simulink model "horn"  (Simulink 7.8)
settings: Solver=ode45  StartTime=0.0  StopTime=1000  RelTol=1e-3
undefined symbols (not defined in the file): magnitude
libraries: simulink x8
settings Model: Creator=ranasa1  LastModifiedBy=ranasa1

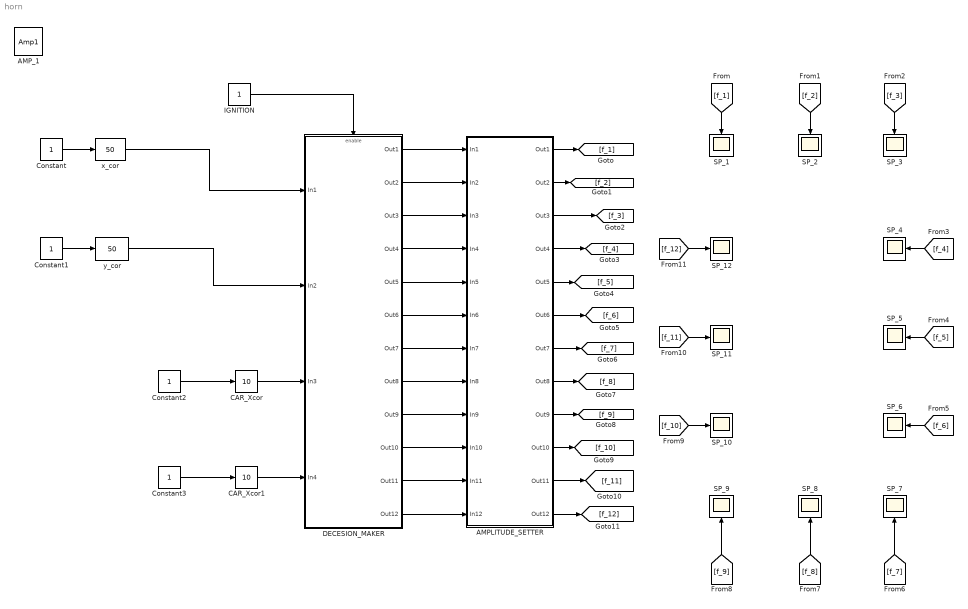
== system horn ==
  AMPLITUDE_SETTER : Subsystem  TreatAsAtomicUnit=on
      settings: RTWFcnNameOpts=Use subsystem name  RTWFileNameOpts=Use function name
  AMP_1 : DataStoreMemory  DataStoreName=Amp1  ReadBeforeWriteMsg=warning  WriteAfterWriteMsg=warning  WriteAfterReadMsg=warning  mask(TL_DataStoreMemory){data={'date',736152.61579912039}}
      settings: CopyFcn=if exist('tl_reset_reviewflag') == 2, tl_reset_reviewflag(gcbh); end  DeleteFcn=if exist('delete_tlblock','file')==2,delete_tlblock(gcbh);end  NameChangeFcn=if exist('rename_tlblock','file')==2,rename_tlblock(gcbh);end  OpenFcn=if exist('tl_open_blockdlg','file')==2,tl_open_blockdlg(gcbh);else,open_system(gcbh,'parameter');end
      mask Help: eval(['if exist(''tl_online_help'',''file'') == 2, tl_online_help(''Topic'',''TL_DataStoreMemory''),else, web([''jar:file:///'',matlabroot,''/help/toolbox/simulink/help.jar!/slref/' lower(get_param(gcbh,'Blocktype')) '.html''], ''-helpbrowser''),end'])
      mask Display: plot([-0.05, 1.05, NaN, -0.05, 1.05],[.01, .01, NaN, .99, .99])
  CAR_Xcor : simulink/Math Operations/Slider Gain  low=0  gain=10  high=20
  CAR_Xcor1 : simulink/Math Operations/Slider Gain  low=0  gain=10  high=20
  Constant{,1..3} (4 alike) : Constant
  DECESION_MAKER : Subsystem  TreatAsAtomicUnit=on
      settings: RTWFcnNameOpts=Use subsystem name  RTWFileNameOpts=Use function name
  IGNITION : Constant
  SP_{1..12} (12 alike) : Scope
      SP_10 settings: SaveName=ScopeData10
      SP_11 settings: SaveName=ScopeData11
      SP_12 settings: SaveName=ScopeData12
      SP_2 settings: SaveName=ScopeData2
      SP_3 settings: SaveName=ScopeData3
      SP_4 settings: SaveName=ScopeData4
      SP_5 settings: SaveName=ScopeData5
      SP_6 settings: SaveName=ScopeData6
      SP_7 settings: SaveName=ScopeData7
      SP_8 settings: SaveName=ScopeData8
      SP_9 settings: SaveName=ScopeData9
  x_cor : simulink/Math Operations/Slider Gain  low=0  gain=50  high=50
  y_cor : simulink/Math Operations/Slider Gain  low=0  gain=50  high=50
  wires:
  DECESION_MAKER/1(Out1) -> AMPLITUDE_SETTER/1(In1)
  DECESION_MAKER/2(Out2) -> AMPLITUDE_SETTER/2(In2)
  DECESION_MAKER/3(Out3) -> AMPLITUDE_SETTER/3(In3)
  DECESION_MAKER/4(Out4) -> AMPLITUDE_SETTER/4(In4)
  DECESION_MAKER/5(Out5) -> AMPLITUDE_SETTER/5(In5)
  DECESION_MAKER/6(Out6) -> AMPLITUDE_SETTER/6(In6)
  DECESION_MAKER/7(Out7) -> AMPLITUDE_SETTER/7(In7)
  DECESION_MAKER/8(Out8) -> AMPLITUDE_SETTER/8(In8)
  DECESION_MAKER/9(Out9) -> AMPLITUDE_SETTER/9(In9)
  DECESION_MAKER/10(Out10) -> AMPLITUDE_SETTER/10(In10)
  DECESION_MAKER/11(Out11) -> AMPLITUDE_SETTER/11(In11)
  DECESION_MAKER/12(Out12) -> AMPLITUDE_SETTER/12(In12)
  Constant/1 -> x_cor/1
  Constant1/1 -> y_cor/1
  AMPLITUDE_SETTER/1(Out1) -> [f_1]
  AMPLITUDE_SETTER/2(Out2) -> [f_2]
  AMPLITUDE_SETTER/3(Out3) -> [f_3]
  AMPLITUDE_SETTER/4(Out4) -> [f_4]
  AMPLITUDE_SETTER/5(Out5) -> [f_5]
  AMPLITUDE_SETTER/6(Out6) -> [f_6]
  AMPLITUDE_SETTER/7(Out7) -> [f_7]
  AMPLITUDE_SETTER/8(Out8) -> [f_8]
  AMPLITUDE_SETTER/9(Out9) -> [f_9]
  AMPLITUDE_SETTER/10(Out10) -> [f_10]
  AMPLITUDE_SETTER/11(Out11) -> [f_11]
  AMPLITUDE_SETTER/12(Out12) -> [f_12]
  [f_1] -> SP_1/1
  [f_2] -> SP_2/1
  [f_3] -> SP_3/1
  [f_4] -> SP_4/1
  [f_5] -> SP_5/1
  [f_6] -> SP_6/1
  [f_7] -> SP_7/1
  [f_8] -> SP_8/1
  [f_9] -> SP_9/1
  [f_10] -> SP_10/1
  [f_11] -> SP_11/1
  [f_12] -> SP_12/1
  Constant2/1 -> CAR_Xcor/1
  CAR_Xcor/1 -> DECESION_MAKER/3(In3)
  Constant3/1 -> CAR_Xcor1/1
  CAR_Xcor1/1 -> DECESION_MAKER/4(In4)
  x_cor/1 -> DECESION_MAKER/1(In1)
  y_cor/1 -> DECESION_MAKER/2(In2)
  IGNITION/1 -> DECESION_MAKER/Enable

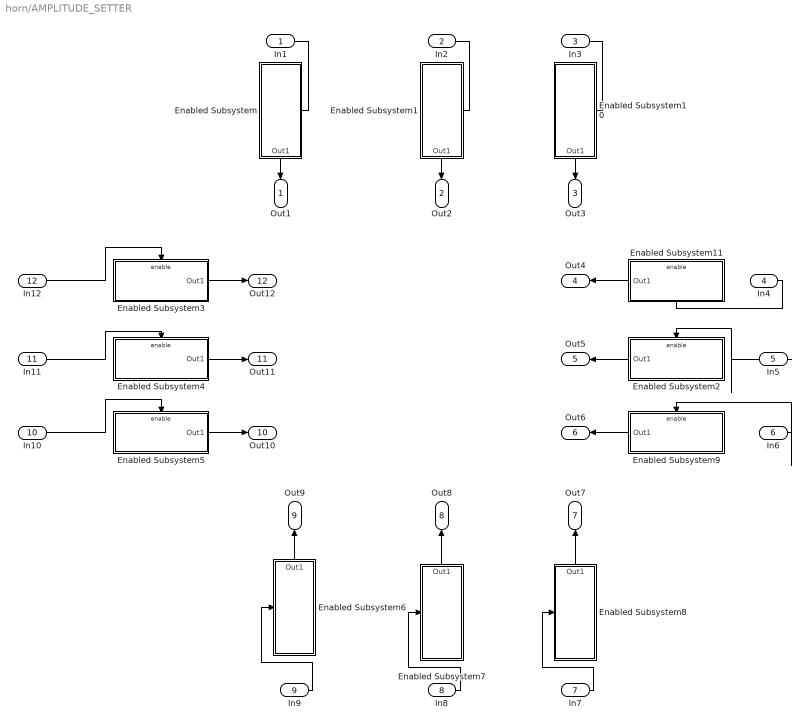
== system horn/AMPLITUDE_SETTER ==
  In1 : Inport
  In2 : Inport  Port=2
  In3 : Inport  Port=3
  In4 : Inport  Port=4
  In5 : Inport  Port=5
  In6 : Inport  Port=6
  In7 : Inport  Port=7
  In8 : Inport  Port=8
  In9 : Inport  Port=9
  In10 : Inport  Port=10
  In11 : Inport  Port=11
  In12 : Inport  Port=12
  Enabled Subsystem : Subsystem  TreatAsAtomicUnit=on
  Enabled Subsystem1 : Subsystem  TreatAsAtomicUnit=on
  Enabled Subsystem10 : Subsystem  TreatAsAtomicUnit=on
  Enabled Subsystem11 : Subsystem  TreatAsAtomicUnit=on
  Enabled Subsystem2 : Subsystem  TreatAsAtomicUnit=on
  Enabled Subsystem3 : Subsystem  TreatAsAtomicUnit=on
  Enabled Subsystem4 : Subsystem  TreatAsAtomicUnit=on
  Enabled Subsystem5 : Subsystem  TreatAsAtomicUnit=on
  Enabled Subsystem6 : Subsystem  TreatAsAtomicUnit=on
  Enabled Subsystem7 : Subsystem  TreatAsAtomicUnit=on
  Enabled Subsystem8 : Subsystem  TreatAsAtomicUnit=on
  Enabled Subsystem9 : Subsystem  TreatAsAtomicUnit=on
  Out1 : Outport
  Out2 : Outport  Port=2
  Out3 : Outport  Port=3
  Out4 : Outport  Port=4
  Out5 : Outport  Port=5
  Out6 : Outport  Port=6
  Out7 : Outport  Port=7
  Out8 : Outport  Port=8
  Out9 : Outport  Port=9
  Out10 : Outport  Port=10
  Out11 : Outport  Port=11
  Out12 : Outport  Port=12
  wires:
  Enabled Subsystem/1(Out1) -> Out1/1
  Enabled Subsystem1/1(Out1) -> Out2/1
  Enabled Subsystem10/1(Out1) -> Out3/1
  Enabled Subsystem11/1(Out1) -> Out4/1
  Enabled Subsystem2/1(Out1) -> Out5/1
  Enabled Subsystem9/1(Out1) -> Out6/1
  Enabled Subsystem8/1(Out1) -> Out7/1
  Enabled Subsystem6/1(Out1) -> Out9/1
  Enabled Subsystem7/1(Out1) -> Out8/1
  Enabled Subsystem3/1(Out1) -> Out12/1
  Enabled Subsystem4/1(Out1) -> Out11/1
  Enabled Subsystem5/1(Out1) -> Out10/1
  In1/1 -> Enabled Subsystem/Enable
  In2/1 -> Enabled Subsystem1/Enable
  In3/1 -> Enabled Subsystem10/Enable
  In4/1 -> Enabled Subsystem11/Enable
  In5/1 -> Enabled Subsystem2/Enable
  In6/1 -> Enabled Subsystem9/Enable
  In7/1 -> Enabled Subsystem8/Enable
  In8/1 -> Enabled Subsystem7/Enable
  In9/1 -> Enabled Subsystem6/Enable
  In10/1 -> Enabled Subsystem5/Enable
  In11/1 -> Enabled Subsystem4/Enable
  In12/1 -> Enabled Subsystem3/Enable

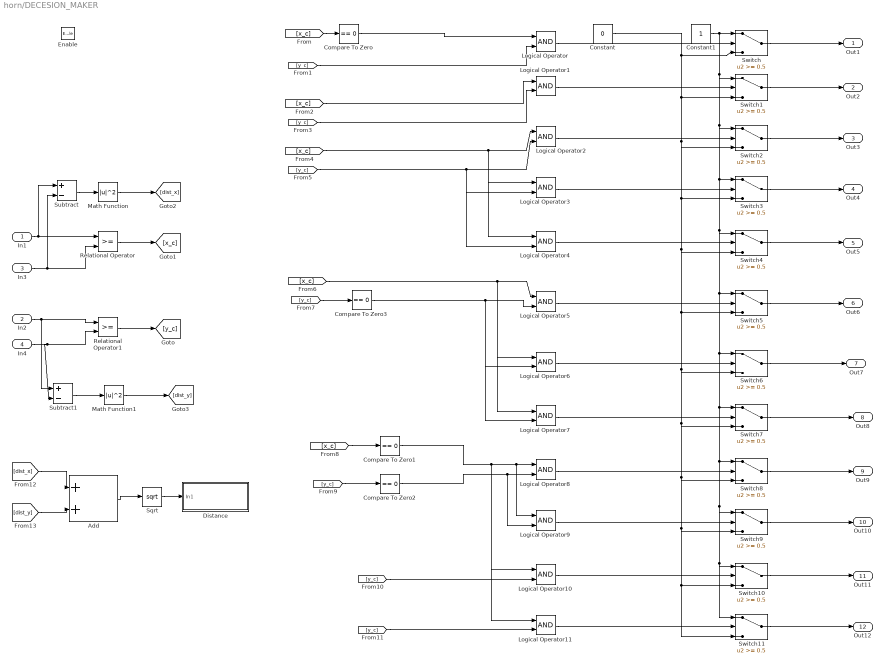
== system horn/DECESION_MAKER ==
  In1 : Inport
  In2 : Inport  Port=2
  In3 : Inport  Port=3
  In4 : Inport  Port=4
  Enable : EnablePort
  Add : Sum
  Compare To Zero{,1..3} (4 alike) : simulink/Logic and Bit Operations/Compare To Zero  relop===  OutDataTypeStr=uint8
  Constant : Constant  Value=0
  Constant1 : Constant
  Distance : Subsystem  TreatAsAtomicUnit=on
      settings: RTWFcnNameOpts=Use subsystem name  RTWFileNameOpts=Use function name
  Logical Operator{,1..11} (12 alike) : Logic  AllPortsSameDT=off  OutDataTypeStr=boolean
  Math Function : Math  Operator=magnitude^2  SaturateOnIntegerOverflow=on
  Math Function1 : Math  Operator=magnitude^2  SaturateOnIntegerOverflow=on
  Relational Operator : RelationalOperator  OutDataTypeStr=boolean
  Relational Operator1 : RelationalOperator  OutDataTypeStr=boolean
  Sqrt : Sqrt  SaturateOnIntegerOverflow=on
  Subtract : Sum  Inputs=+-
  Subtract1 : Sum  Inputs=+-
  Switch{,1..11} (12 alike) : Switch  Threshold=0.5
  Out1 : Outport
  Out2 : Outport  Port=2
  Out3 : Outport  Port=3
  Out4 : Outport  Port=4
  Out5 : Outport  Port=5
  Out6 : Outport  Port=6
  Out7 : Outport  Port=7
  Out8 : Outport  Port=8
  Out9 : Outport  Port=9
  Out10 : Outport  Port=10
  Out11 : Outport  Port=11
  Out12 : Outport  Port=12
  wires:
  Switch/1 -> Out1/1
  Switch1/1 -> Out2/1
  Switch2/1 -> Out3/1
  Switch3/1 -> Out4/1
  Switch4/1 -> Out5/1
  Switch5/1 -> Out6/1
  Switch6/1 -> Out7/1
  Switch7/1 -> Out8/1
  Switch8/1 -> Out9/1
  Switch9/1 -> Out10/1
  Switch10/1 -> Out11/1
  Switch11/1 -> Out12/1
  In1/1 -> Relational Operator/1, Subtract/1
  In3/1 -> Relational Operator/2, Subtract/2
  In2/1 -> Relational Operator1/1, Subtract1/1
  In4/1 -> Relational Operator1/2, Subtract1/2
  Relational Operator/1 -> [x_c]
  Relational Operator1/1 -> [y_c]
  Logical Operator/1 -> Switch/2
  Logical Operator1/1 -> Switch1/2
  Logical Operator2/1 -> Switch2/2
  Logical Operator3/1 -> Switch3/2
  Logical Operator4/1 -> Switch4/2
  Logical Operator5/1 -> Switch5/2
  Logical Operator6/1 -> Switch6/2
  Logical Operator7/1 -> Switch7/2
  Logical Operator8/1 -> Switch8/2
  Logical Operator9/1 -> Switch9/2
  Logical Operator10/1 -> Switch10/2
  Logical Operator11/1 -> Switch11/2
  [x_c] -> Compare To Zero/1
  [y_c] -> Logical Operator1/2
  [x_c] -> Logical Operator1/1
  [x_c] -> Logical Operator2/1, Logical Operator3/1, Logical Operator4/1
  [y_c] -> Logical Operator2/2, Logical Operator3/2, Logical Operator4/2
  [y_c] -> Compare To Zero3/1
  [x_c] -> Logical Operator5/1, Logical Operator6/1, Logical Operator7/1
  Compare To Zero3/1 -> Logical Operator5/2, Logical Operator6/2, Logical Operator7/2
  Constant1/1 -> Switch/1, Switch1/1, Switch2/1, Switch3/1, Switch4/1, Switch5/1, Switch6/1, Switch7/1, Switch8/1, Switch9/1, Switch10/1, Switch11/1
  Constant/1 -> Switch/3, Switch1/3, Switch2/3, Switch3/3, Switch4/3, Switch5/3, Switch6/3, Switch7/3, Switch8/3, Switch9/3, Switch10/3, Switch11/3
  [y_c] -> Logical Operator/2
  Compare To Zero/1 -> Logical Operator/1
  [x_c] -> Compare To Zero1/1
  [y_c] -> Compare To Zero2/1
  Compare To Zero1/1 -> Logical Operator8/1, Logical Operator9/1, Logical Operator10/1, Logical Operator11/1
  Compare To Zero2/1 -> Logical Operator8/2, Logical Operator9/2
  [y_c] -> Logical Operator10/2
  [y_c] -> Logical Operator11/2
  Subtract/1 -> Math Function/1
  Subtract1/1 -> Math Function1/1
  Math Function/1 -> [dist_x]
  Math Function1/1 -> [dist_y]
  [dist_x] -> Add/1
  [dist_y] -> Add/2
  Add/1 -> Sqrt/1
  Sqrt/1 -> Distance/1(In1)

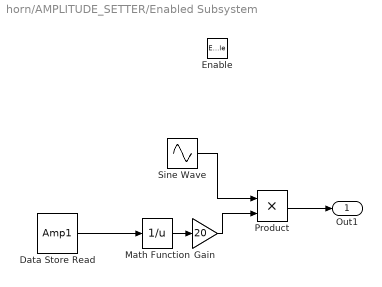
== system horn/AMPLITUDE_SETTER/Enabled Subsystem ==
  Enable : EnablePort
  Data Store Read : DataStoreRead  DataStoreName=Amp1  mask(TL_DataStoreRead){data={'date',736152.73192049772}}
      settings: DeleteFcn=if exist('delete_tlblock','file')==2,delete_tlblock(gcbh);end  NameChangeFcn=if exist('rename_tlblock','file')==2,rename_tlblock(gcbh);end  OpenFcn=if exist('tl_open_blockdlg','file')==2,tl_open_blockdlg(gcbh);else,open_system(gcbh,'parameter');end
      mask Help: eval(['if exist(''tl_online_help'',''file'') == 2, tl_online_help(''Topic'',''TL_DataStoreRead''),else, web([''jar:file:///'',matlabroot,''/help/toolbox/simulink/help.jar!/slref/' lower(get_param(gcbh,'Blocktype')) '.html''], ''-helpbrowser''),end'])
      mask Display: plot([-0.05, 1.05, NaN, -0.05, 1.05],[.01, .01, NaN, .99, .99])
  Gain : Gain  Gain=20
  Math Function : Math  Operator=reciprocal  SaturateOnIntegerOverflow=on
  Product : Product  RndMeth=Zero
  Sine Wave : Sin  SampleTime=0
  Out1 : Outport
  wires:
  Data Store Read/1 -> Math Function/1
  Sine Wave/1 -> Product/1
  Product/1 -> Out1/1
  Math Function/1 -> Gain/1
  Gain/1 -> Product/2

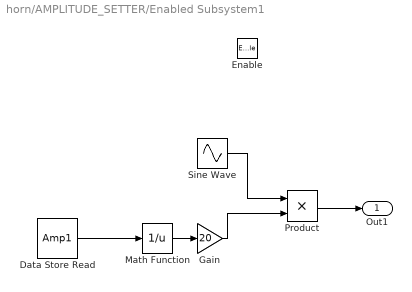
== system horn/AMPLITUDE_SETTER/Enabled Subsystem1 ==
  Enable : EnablePort
  Data Store Read : DataStoreRead  DataStoreName=Amp1  mask(TL_DataStoreRead){data={'date',736152.75838344905}}
      settings: DeleteFcn=if exist('delete_tlblock','file')==2,delete_tlblock(gcbh);end  NameChangeFcn=if exist('rename_tlblock','file')==2,rename_tlblock(gcbh);end  OpenFcn=if exist('tl_open_blockdlg','file')==2,tl_open_blockdlg(gcbh);else,open_system(gcbh,'parameter');end
      mask Help: eval(['if exist(''tl_online_help'',''file'') == 2, tl_online_help(''Topic'',''TL_DataStoreRead''),else, web([''jar:file:///'',matlabroot,''/help/toolbox/simulink/help.jar!/slref/' lower(get_param(gcbh,'Blocktype')) '.html''], ''-helpbrowser''),end'])
      mask Display: plot([-0.05, 1.05, NaN, -0.05, 1.05],[.01, .01, NaN, .99, .99])
  Gain : Gain  Gain=20
  Math Function : Math  Operator=reciprocal  SaturateOnIntegerOverflow=on
  Product : Product  RndMeth=Zero
  Sine Wave : Sin  SampleTime=0
  Out1 : Outport
  wires:
  Product/1 -> Out1/1
  Sine Wave/1 -> Product/1
  Data Store Read/1 -> Math Function/1
  Math Function/1 -> Gain/1
  Gain/1 -> Product/2

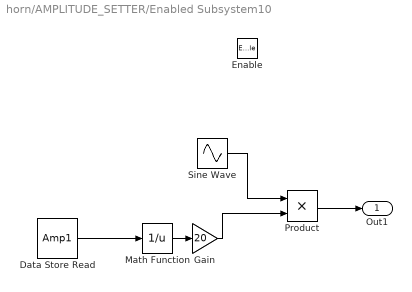
== system horn/AMPLITUDE_SETTER/Enabled Subsystem10 ==
  Enable : EnablePort
  Data Store Read : DataStoreRead  DataStoreName=Amp1  mask(TL_DataStoreRead){data={'date',736152.73192049772}}
      settings: DeleteFcn=if exist('delete_tlblock','file')==2,delete_tlblock(gcbh);end  NameChangeFcn=if exist('rename_tlblock','file')==2,rename_tlblock(gcbh);end  OpenFcn=if exist('tl_open_blockdlg','file')==2,tl_open_blockdlg(gcbh);else,open_system(gcbh,'parameter');end
      mask Help: eval(['if exist(''tl_online_help'',''file'') == 2, tl_online_help(''Topic'',''TL_DataStoreRead''),else, web([''jar:file:///'',matlabroot,''/help/toolbox/simulink/help.jar!/slref/' lower(get_param(gcbh,'Blocktype')) '.html''], ''-helpbrowser''),end'])
      mask Display: plot([-0.05, 1.05, NaN, -0.05, 1.05],[.01, .01, NaN, .99, .99])
  Gain : Gain  Gain=20
  Math Function : Math  Operator=reciprocal  SaturateOnIntegerOverflow=on
  Product : Product  RndMeth=Zero
  Sine Wave : Sin  SampleTime=0
  Out1 : Outport
  wires:
  Sine Wave/1 -> Product/1
  Product/1 -> Out1/1
  Data Store Read/1 -> Math Function/1
  Math Function/1 -> Gain/1
  Gain/1 -> Product/2

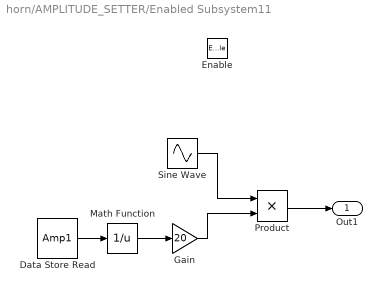
== system horn/AMPLITUDE_SETTER/Enabled Subsystem11 ==
  Enable : EnablePort
  Data Store Read : DataStoreRead  DataStoreName=Amp1  mask(TL_DataStoreRead){data={'date',736152.73192049772}}
      settings: DeleteFcn=if exist('delete_tlblock','file')==2,delete_tlblock(gcbh);end  NameChangeFcn=if exist('rename_tlblock','file')==2,rename_tlblock(gcbh);end  OpenFcn=if exist('tl_open_blockdlg','file')==2,tl_open_blockdlg(gcbh);else,open_system(gcbh,'parameter');end
      mask Help: eval(['if exist(''tl_online_help'',''file'') == 2, tl_online_help(''Topic'',''TL_DataStoreRead''),else, web([''jar:file:///'',matlabroot,''/help/toolbox/simulink/help.jar!/slref/' lower(get_param(gcbh,'Blocktype')) '.html''], ''-helpbrowser''),end'])
      mask Display: plot([-0.05, 1.05, NaN, -0.05, 1.05],[.01, .01, NaN, .99, .99])
  Gain : Gain  Gain=20
  Math Function : Math  Operator=reciprocal  SaturateOnIntegerOverflow=on
  Product : Product  RndMeth=Zero
  Sine Wave : Sin  SampleTime=0
  Out1 : Outport
  wires:
  Product/1 -> Out1/1
  Sine Wave/1 -> Product/1
  Data Store Read/1 -> Math Function/1
  Math Function/1 -> Gain/1
  Gain/1 -> Product/2

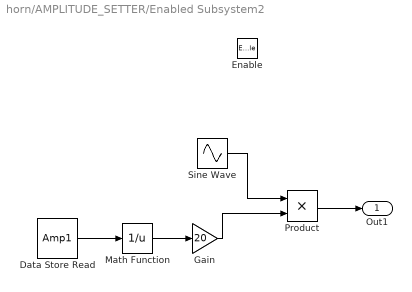
== system horn/AMPLITUDE_SETTER/Enabled Subsystem2 ==
  Enable : EnablePort
  Data Store Read : DataStoreRead  DataStoreName=Amp1  mask(TL_DataStoreRead){data={'date',736152.73192049772}}
      settings: DeleteFcn=if exist('delete_tlblock','file')==2,delete_tlblock(gcbh);end  NameChangeFcn=if exist('rename_tlblock','file')==2,rename_tlblock(gcbh);end  OpenFcn=if exist('tl_open_blockdlg','file')==2,tl_open_blockdlg(gcbh);else,open_system(gcbh,'parameter');end
      mask Help: eval(['if exist(''tl_online_help'',''file'') == 2, tl_online_help(''Topic'',''TL_DataStoreRead''),else, web([''jar:file:///'',matlabroot,''/help/toolbox/simulink/help.jar!/slref/' lower(get_param(gcbh,'Blocktype')) '.html''], ''-helpbrowser''),end'])
      mask Display: plot([-0.05, 1.05, NaN, -0.05, 1.05],[.01, .01, NaN, .99, .99])
  Gain : Gain  Gain=20
  Math Function : Math  Operator=reciprocal  SaturateOnIntegerOverflow=on
  Product : Product  RndMeth=Zero
  Sine Wave : Sin  SampleTime=0
  Out1 : Outport
  wires:
  Sine Wave/1 -> Product/1
  Product/1 -> Out1/1
  Data Store Read/1 -> Math Function/1
  Math Function/1 -> Gain/1
  Gain/1 -> Product/2

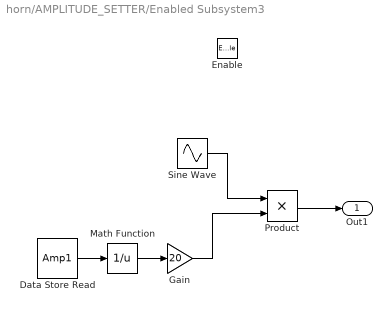
== system horn/AMPLITUDE_SETTER/Enabled Subsystem3 ==
  Enable : EnablePort
  Data Store Read : DataStoreRead  DataStoreName=Amp1  mask(TL_DataStoreRead){data={'date',736152.73192049772}}
      settings: DeleteFcn=if exist('delete_tlblock','file')==2,delete_tlblock(gcbh);end  NameChangeFcn=if exist('rename_tlblock','file')==2,rename_tlblock(gcbh);end  OpenFcn=if exist('tl_open_blockdlg','file')==2,tl_open_blockdlg(gcbh);else,open_system(gcbh,'parameter');end
      mask Help: eval(['if exist(''tl_online_help'',''file'') == 2, tl_online_help(''Topic'',''TL_DataStoreRead''),else, web([''jar:file:///'',matlabroot,''/help/toolbox/simulink/help.jar!/slref/' lower(get_param(gcbh,'Blocktype')) '.html''], ''-helpbrowser''),end'])
      mask Display: plot([-0.05, 1.05, NaN, -0.05, 1.05],[.01, .01, NaN, .99, .99])
  Gain : Gain  Gain=20
  Math Function : Math  Operator=reciprocal  SaturateOnIntegerOverflow=on
  Product : Product  RndMeth=Zero
  Sine Wave : Sin  SampleTime=0
  Out1 : Outport
  wires:
  Product/1 -> Out1/1
  Sine Wave/1 -> Product/1
  Data Store Read/1 -> Math Function/1
  Math Function/1 -> Gain/1
  Gain/1 -> Product/2

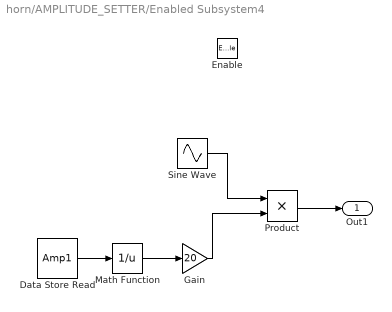
== system horn/AMPLITUDE_SETTER/Enabled Subsystem4 ==
  Enable : EnablePort
  Data Store Read : DataStoreRead  DataStoreName=Amp1  mask(TL_DataStoreRead){data={'date',736152.73192049772}}
      settings: DeleteFcn=if exist('delete_tlblock','file')==2,delete_tlblock(gcbh);end  NameChangeFcn=if exist('rename_tlblock','file')==2,rename_tlblock(gcbh);end  OpenFcn=if exist('tl_open_blockdlg','file')==2,tl_open_blockdlg(gcbh);else,open_system(gcbh,'parameter');end
      mask Help: eval(['if exist(''tl_online_help'',''file'') == 2, tl_online_help(''Topic'',''TL_DataStoreRead''),else, web([''jar:file:///'',matlabroot,''/help/toolbox/simulink/help.jar!/slref/' lower(get_param(gcbh,'Blocktype')) '.html''], ''-helpbrowser''),end'])
      mask Display: plot([-0.05, 1.05, NaN, -0.05, 1.05],[.01, .01, NaN, .99, .99])
  Gain : Gain  Gain=20
  Math Function : Math  Operator=reciprocal  SaturateOnIntegerOverflow=on
  Product : Product  RndMeth=Zero
  Sine Wave : Sin  SampleTime=0
  Out1 : Outport
  wires:
  Sine Wave/1 -> Product/1
  Product/1 -> Out1/1
  Data Store Read/1 -> Math Function/1
  Math Function/1 -> Gain/1
  Gain/1 -> Product/2

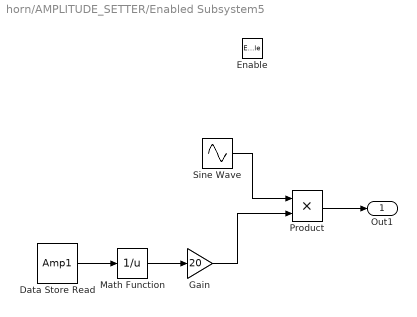
== system horn/AMPLITUDE_SETTER/Enabled Subsystem5 ==
  Enable : EnablePort
  Data Store Read : DataStoreRead  DataStoreName=Amp1  mask(TL_DataStoreRead){data={'date',736152.73192049772}}
      settings: DeleteFcn=if exist('delete_tlblock','file')==2,delete_tlblock(gcbh);end  NameChangeFcn=if exist('rename_tlblock','file')==2,rename_tlblock(gcbh);end  OpenFcn=if exist('tl_open_blockdlg','file')==2,tl_open_blockdlg(gcbh);else,open_system(gcbh,'parameter');end
      mask Help: eval(['if exist(''tl_online_help'',''file'') == 2, tl_online_help(''Topic'',''TL_DataStoreRead''),else, web([''jar:file:///'',matlabroot,''/help/toolbox/simulink/help.jar!/slref/' lower(get_param(gcbh,'Blocktype')) '.html''], ''-helpbrowser''),end'])
      mask Display: plot([-0.05, 1.05, NaN, -0.05, 1.05],[.01, .01, NaN, .99, .99])
  Gain : Gain  Gain=20
  Math Function : Math  Operator=reciprocal  SaturateOnIntegerOverflow=on
  Product : Product  RndMeth=Zero
  Sine Wave : Sin  SampleTime=0
  Out1 : Outport
  wires:
  Product/1 -> Out1/1
  Sine Wave/1 -> Product/1
  Data Store Read/1 -> Math Function/1
  Math Function/1 -> Gain/1
  Gain/1 -> Product/2

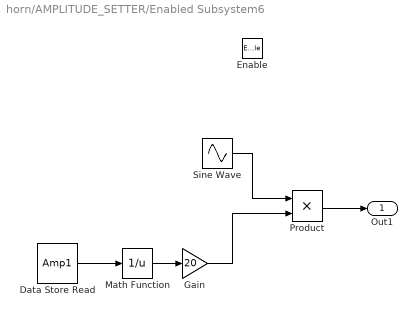
== system horn/AMPLITUDE_SETTER/Enabled Subsystem6 ==
  Enable : EnablePort
  Data Store Read : DataStoreRead  DataStoreName=Amp1  mask(TL_DataStoreRead){data={'date',736152.73192049772}}
      settings: DeleteFcn=if exist('delete_tlblock','file')==2,delete_tlblock(gcbh);end  NameChangeFcn=if exist('rename_tlblock','file')==2,rename_tlblock(gcbh);end  OpenFcn=if exist('tl_open_blockdlg','file')==2,tl_open_blockdlg(gcbh);else,open_system(gcbh,'parameter');end
      mask Help: eval(['if exist(''tl_online_help'',''file'') == 2, tl_online_help(''Topic'',''TL_DataStoreRead''),else, web([''jar:file:///'',matlabroot,''/help/toolbox/simulink/help.jar!/slref/' lower(get_param(gcbh,'Blocktype')) '.html''], ''-helpbrowser''),end'])
      mask Display: plot([-0.05, 1.05, NaN, -0.05, 1.05],[.01, .01, NaN, .99, .99])
  Gain : Gain  Gain=20
  Math Function : Math  Operator=reciprocal  SaturateOnIntegerOverflow=on
  Product : Product  RndMeth=Zero
  Sine Wave : Sin  SampleTime=0
  Out1 : Outport
  wires:
  Sine Wave/1 -> Product/1
  Product/1 -> Out1/1
  Data Store Read/1 -> Math Function/1
  Math Function/1 -> Gain/1
  Gain/1 -> Product/2

== system horn/AMPLITUDE_SETTER/Enabled Subsystem7 ==
  Enable : EnablePort
  Data Store Read : DataStoreRead  DataStoreName=Amp1  mask(TL_DataStoreRead){data={'date',736152.73192049772}}
      settings: DeleteFcn=if exist('delete_tlblock','file')==2,delete_tlblock(gcbh);end  NameChangeFcn=if exist('rename_tlblock','file')==2,rename_tlblock(gcbh);end  OpenFcn=if exist('tl_open_blockdlg','file')==2,tl_open_blockdlg(gcbh);else,open_system(gcbh,'parameter');end
      mask Help: eval(['if exist(''tl_online_help'',''file'') == 2, tl_online_help(''Topic'',''TL_DataStoreRead''),else, web([''jar:file:///'',matlabroot,''/help/toolbox/simulink/help.jar!/slref/' lower(get_param(gcbh,'Blocktype')) '.html''], ''-helpbrowser''),end'])
      mask Display: plot([-0.05, 1.05, NaN, -0.05, 1.05],[.01, .01, NaN, .99, .99])
  Gain : Gain  Gain=20
  Math Function : Math  Operator=reciprocal  SaturateOnIntegerOverflow=on
  Product : Product  RndMeth=Zero
  Sine Wave : Sin  SampleTime=0
  Out1 : Outport
  wires:
  Product/1 -> Out1/1
  Sine Wave/1 -> Product/1
  Data Store Read/1 -> Math Function/1
  Math Function/1 -> Gain/1
  Gain/1 -> Product/2

== system horn/AMPLITUDE_SETTER/Enabled Subsystem8 ==
  Enable : EnablePort
  Data Store Read : DataStoreRead  DataStoreName=Amp1  mask(TL_DataStoreRead){data={'date',736152.73192049772}}
      settings: DeleteFcn=if exist('delete_tlblock','file')==2,delete_tlblock(gcbh);end  NameChangeFcn=if exist('rename_tlblock','file')==2,rename_tlblock(gcbh);end  OpenFcn=if exist('tl_open_blockdlg','file')==2,tl_open_blockdlg(gcbh);else,open_system(gcbh,'parameter');end
      mask Help: eval(['if exist(''tl_online_help'',''file'') == 2, tl_online_help(''Topic'',''TL_DataStoreRead''),else, web([''jar:file:///'',matlabroot,''/help/toolbox/simulink/help.jar!/slref/' lower(get_param(gcbh,'Blocktype')) '.html''], ''-helpbrowser''),end'])
      mask Display: plot([-0.05, 1.05, NaN, -0.05, 1.05],[.01, .01, NaN, .99, .99])
  Gain : Gain  Gain=20
  Math Function : Math  Operator=reciprocal  SaturateOnIntegerOverflow=on
  Product : Product  RndMeth=Zero
  Sine Wave : Sin  SampleTime=0
  Out1 : Outport
  wires:
  Sine Wave/1 -> Product/1
  Product/1 -> Out1/1
  Data Store Read/1 -> Math Function/1
  Math Function/1 -> Gain/1
  Gain/1 -> Product/2

== system horn/AMPLITUDE_SETTER/Enabled Subsystem9 ==
  Enable : EnablePort
  Data Store Read : DataStoreRead  DataStoreName=Amp1  mask(TL_DataStoreRead){data={'date',736152.73192049772}}
      settings: DeleteFcn=if exist('delete_tlblock','file')==2,delete_tlblock(gcbh);end  NameChangeFcn=if exist('rename_tlblock','file')==2,rename_tlblock(gcbh);end  OpenFcn=if exist('tl_open_blockdlg','file')==2,tl_open_blockdlg(gcbh);else,open_system(gcbh,'parameter');end
      mask Help: eval(['if exist(''tl_online_help'',''file'') == 2, tl_online_help(''Topic'',''TL_DataStoreRead''),else, web([''jar:file:///'',matlabroot,''/help/toolbox/simulink/help.jar!/slref/' lower(get_param(gcbh,'Blocktype')) '.html''], ''-helpbrowser''),end'])
      mask Display: plot([-0.05, 1.05, NaN, -0.05, 1.05],[.01, .01, NaN, .99, .99])
  Gain : Gain  Gain=20
  Math Function : Math  Operator=reciprocal  SaturateOnIntegerOverflow=on
  Product : Product  RndMeth=Zero
  Sine Wave : Sin  SampleTime=0
  Out1 : Outport
  wires:
  Product/1 -> Out1/1
  Sine Wave/1 -> Product/1
  Data Store Read/1 -> Math Function/1
  Math Function/1 -> Gain/1
  Gain/1 -> Product/2

== system horn/DECESION_MAKER/Distance ==
  In1 : Inport
  Data Store Write : DataStoreWrite  DataStoreName=Amp1  mask(TL_DataStoreWrite){data={'date',736152.73031916667}}
      settings: DeleteFcn=if exist('delete_tlblock','file')==2,delete_tlblock(gcbh);end  NameChangeFcn=if exist('rename_tlblock','file')==2,rename_tlblock(gcbh);end  OpenFcn=if exist('tl_open_blockdlg','file')==2,tl_open_blockdlg(gcbh);else,open_system(gcbh,'parameter');end
      mask Help: eval(['if exist(''tl_online_help'',''file'') == 2, tl_online_help(''Topic'',''TL_DataStoreWrite''),else, web([''jar:file:///'',matlabroot,''/help/toolbox/simulink/help.jar!/slref/' lower(get_param(gcbh,'Blocktype')) '.html''], ''-helpbrowser''),end'])
      mask Display: plot([-0.05, 1.05, NaN, -0.05, 1.05],[.01, .01, NaN, .99, .99])
  wires:
  In1/1 -> Data Store Write/1
